simulink model "TST_EISGov_Governor"  (R2016b)
settings: Solver=FixedStepDiscrete  StartTime=0.0  StopTime=simTime  FixedStep=sampleTime  RelTol=1e-3
values from neighbouring files (symbols this model uses):
  testCase = 1    [initTST_EISGov_Governor_001.m]    (also in initTST_EISGov_Governor_002.m = 2; initTST_EISGov_Governor_003.m = 3; initTST_EISGov_Governor_004.m = 4; initTST_EISGov_Governor_005.m = 5)
libraries: simulink x43, UnitTest_Lib x36
(part 3 of 4)

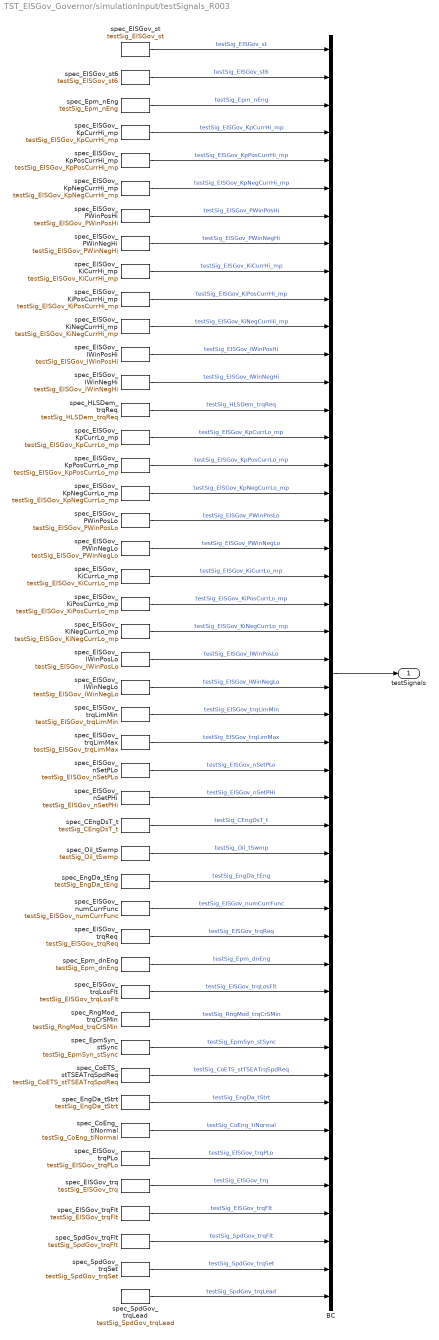
== system TST_EISGov_Governor/simulationInput/testSignals_R003 ==
  BC : BusCreator  Inputs=46
  spec_CEngDsT_t : FromWorkspace  VariableName=testSig_CEngDsT_t  Interpolate=off  OutputAfterFinalValue=Holding final value
  spec_CoETS_stTSEATrqSpdReq : FromWorkspace  VariableName=testSig_CoETS_stTSEATrqSpdReq  Interpolate=off  OutputAfterFinalValue=Holding final value
  spec_CoEng_tiNormal : FromWorkspace  VariableName=testSig_CoEng_tiNormal  Interpolate=off  OutputAfterFinalValue=Holding final value
  spec_EISGov_IWinNegHi : FromWorkspace  VariableName=testSig_EISGov_IWinNegHi  Interpolate=off  OutputAfterFinalValue=Holding final value
  spec_EISGov_IWinNegLo : FromWorkspace  VariableName=testSig_EISGov_IWinNegLo  Interpolate=off  OutputAfterFinalValue=Holding final value
  spec_EISGov_IWinPosHi : FromWorkspace  VariableName=testSig_EISGov_IWinPosHi  Interpolate=off  OutputAfterFinalValue=Holding final value
  spec_EISGov_IWinPosLo : FromWorkspace  VariableName=testSig_EISGov_IWinPosLo  Interpolate=off  OutputAfterFinalValue=Holding final value
  spec_EISGov_KiCurrHi_mp : FromWorkspace  VariableName=testSig_EISGov_KiCurrHi_mp  Interpolate=off  OutputAfterFinalValue=Holding final value
  spec_EISGov_KiCurrLo_mp : FromWorkspace  VariableName=testSig_EISGov_KiCurrLo_mp  Interpolate=off  OutputAfterFinalValue=Holding final value
  spec_EISGov_KiNegCurrHi_mp : FromWorkspace  VariableName=testSig_EISGov_KiNegCurrHi_mp  Interpolate=off  OutputAfterFinalValue=Holding final value
  spec_EISGov_KiNegCurrLo_mp : FromWorkspace  VariableName=testSig_EISGov_KiNegCurrLo_mp  Interpolate=off  OutputAfterFinalValue=Holding final value
  spec_EISGov_KiPosCurrHi_mp : FromWorkspace  VariableName=testSig_EISGov_KiPosCurrHi_mp  Interpolate=off  OutputAfterFinalValue=Holding final value
  spec_EISGov_KiPosCurrLo_mp : FromWorkspace  VariableName=testSig_EISGov_KiPosCurrLo_mp  Interpolate=off  OutputAfterFinalValue=Holding final value
  spec_EISGov_KpCurrHi_mp : FromWorkspace  VariableName=testSig_EISGov_KpCurrHi_mp  Interpolate=off  OutputAfterFinalValue=Holding final value
  spec_EISGov_KpCurrLo_mp : FromWorkspace  VariableName=testSig_EISGov_KpCurrLo_mp  Interpolate=off  OutputAfterFinalValue=Holding final value
  spec_EISGov_KpNegCurrHi_mp : FromWorkspace  VariableName=testSig_EISGov_KpNegCurrHi_mp  Interpolate=off  OutputAfterFinalValue=Holding final value
  spec_EISGov_KpNegCurrLo_mp : FromWorkspace  VariableName=testSig_EISGov_KpNegCurrLo_mp  Interpolate=off  OutputAfterFinalValue=Holding final value
  spec_EISGov_KpPosCurrHi_mp : FromWorkspace  VariableName=testSig_EISGov_KpPosCurrHi_mp  Interpolate=off  OutputAfterFinalValue=Holding final value
  spec_EISGov_KpPosCurrLo_mp : FromWorkspace  VariableName=testSig_EISGov_KpPosCurrLo_mp  Interpolate=off  OutputAfterFinalValue=Holding final value
  spec_EISGov_PWinNegHi : FromWorkspace  VariableName=testSig_EISGov_PWinNegHi  Interpolate=off  OutputAfterFinalValue=Holding final value
  spec_EISGov_PWinNegLo : FromWorkspace  VariableName=testSig_EISGov_PWinNegLo  Interpolate=off  OutputAfterFinalValue=Holding final value
  spec_EISGov_PWinPosHi : FromWorkspace  VariableName=testSig_EISGov_PWinPosHi  Interpolate=off  OutputAfterFinalValue=Holding final value
  spec_EISGov_PWinPosLo : FromWorkspace  VariableName=testSig_EISGov_PWinPosLo  Interpolate=off  OutputAfterFinalValue=Holding final value
  spec_EISGov_nSetPHi : FromWorkspace  VariableName=testSig_EISGov_nSetPHi  Interpolate=off  OutputAfterFinalValue=Holding final value
  spec_EISGov_nSetPLo : FromWorkspace  VariableName=testSig_EISGov_nSetPLo  Interpolate=off  OutputAfterFinalValue=Holding final value
  spec_EISGov_numCurrFunc : FromWorkspace  VariableName=testSig_EISGov_numCurrFunc  Interpolate=off  OutputAfterFinalValue=Holding final value
  spec_EISGov_st : FromWorkspace  VariableName=testSig_EISGov_st  Interpolate=off  OutputAfterFinalValue=Holding final value
  spec_EISGov_st6 : FromWorkspace  VariableName=testSig_EISGov_st6  Interpolate=off  OutputAfterFinalValue=Holding final value
  spec_EISGov_trq : FromWorkspace  VariableName=testSig_EISGov_trq  Interpolate=off  OutputAfterFinalValue=Holding final value
  spec_EISGov_trqFlt : FromWorkspace  VariableName=testSig_EISGov_trqFlt  Interpolate=off  OutputAfterFinalValue=Holding final value
  spec_EISGov_trqLimMax : FromWorkspace  VariableName=testSig_EISGov_trqLimMax  Interpolate=off  OutputAfterFinalValue=Holding final value
  spec_EISGov_trqLimMin : FromWorkspace  VariableName=testSig_EISGov_trqLimMin  Interpolate=off  OutputAfterFinalValue=Holding final value
  spec_EISGov_trqLosFlt : FromWorkspace  VariableName=testSig_EISGov_trqLosFlt  Interpolate=off  OutputAfterFinalValue=Holding final value
  spec_EISGov_trqPLo : FromWorkspace  VariableName=testSig_EISGov_trqPLo  Interpolate=off  OutputAfterFinalValue=Holding final value
  spec_EISGov_trqReq : FromWorkspace  VariableName=testSig_EISGov_trqReq  Interpolate=off  OutputAfterFinalValue=Holding final value
  spec_EngDa_tEng : FromWorkspace  VariableName=testSig_EngDa_tEng  Interpolate=off  OutputAfterFinalValue=Holding final value
  spec_EngDa_tStrt : FromWorkspace  VariableName=testSig_EngDa_tStrt  Interpolate=off  OutputAfterFinalValue=Holding final value
  spec_EpmSyn_stSync : FromWorkspace  VariableName=testSig_EpmSyn_stSync  Interpolate=off  OutputAfterFinalValue=Holding final value
  spec_Epm_dnEng : FromWorkspace  VariableName=testSig_Epm_dnEng  Interpolate=off  OutputAfterFinalValue=Holding final value
  spec_Epm_nEng : FromWorkspace  VariableName=testSig_Epm_nEng  Interpolate=off  OutputAfterFinalValue=Holding final value
  spec_HLSDem_trqReq : FromWorkspace  VariableName=testSig_HLSDem_trqReq  Interpolate=off  OutputAfterFinalValue=Holding final value
  spec_Oil_tSwmp : FromWorkspace  VariableName=testSig_Oil_tSwmp  Interpolate=off  OutputAfterFinalValue=Holding final value
  spec_RngMod_trqCrSMin : FromWorkspace  VariableName=testSig_RngMod_trqCrSMin  Interpolate=off  OutputAfterFinalValue=Holding final value
  spec_SpdGov_trqFlt : FromWorkspace  VariableName=testSig_SpdGov_trqFlt  Interpolate=off  OutputAfterFinalValue=Holding final value
  spec_SpdGov_trqLead : FromWorkspace  VariableName=testSig_SpdGov_trqLead  Interpolate=off  OutputAfterFinalValue=Holding final value
  spec_SpdGov_trqSet : FromWorkspace  VariableName=testSig_SpdGov_trqSet  Interpolate=off  OutputAfterFinalValue=Holding final value
  testSignals : Outport
  wires:
  BC/1 -> testSignals/1
  spec_EISGov_st/1 -> BC/1  "testSig_EISGov_st"
  spec_EISGov_st6/1 -> BC/2  "testSig_EISGov_st6"
  spec_Epm_nEng/1 -> BC/3  "testSig_Epm_nEng"
  spec_EISGov_KpCurrHi_mp/1 -> BC/4  "testSig_EISGov_KpCurrHi_mp"
  spec_EISGov_KpPosCurrHi_mp/1 -> BC/5  "testSig_EISGov_KpPosCurrHi_mp"
  spec_EISGov_KpNegCurrHi_mp/1 -> BC/6  "testSig_EISGov_KpNegCurrHi_mp"
  spec_EISGov_PWinPosHi/1 -> BC/7  "testSig_EISGov_PWinPosHi"
  spec_EISGov_PWinNegHi/1 -> BC/8  "testSig_EISGov_PWinNegHi"
  spec_EISGov_KiCurrHi_mp/1 -> BC/9  "testSig_EISGov_KiCurrHi_mp"
  spec_EISGov_KiPosCurrHi_mp/1 -> BC/10  "testSig_EISGov_KiPosCurrHi_mp"
  spec_EISGov_KiNegCurrHi_mp/1 -> BC/11  "testSig_EISGov_KiNegCurrHi_mp"
  spec_EISGov_IWinPosHi/1 -> BC/12  "testSig_EISGov_IWinPosHi"
  spec_EISGov_IWinNegHi/1 -> BC/13  "testSig_EISGov_IWinNegHi"
  spec_HLSDem_trqReq/1 -> BC/14  "testSig_HLSDem_trqReq"
  spec_EISGov_KpCurrLo_mp/1 -> BC/15  "testSig_EISGov_KpCurrLo_mp"
  spec_EISGov_KpPosCurrLo_mp/1 -> BC/16  "testSig_EISGov_KpPosCurrLo_mp"
  spec_EISGov_KpNegCurrLo_mp/1 -> BC/17  "testSig_EISGov_KpNegCurrLo_mp"
  spec_EISGov_PWinPosLo/1 -> BC/18  "testSig_EISGov_PWinPosLo"
  spec_EISGov_PWinNegLo/1 -> BC/19  "testSig_EISGov_PWinNegLo"
  spec_EISGov_KiCurrLo_mp/1 -> BC/20  "testSig_EISGov_KiCurrLo_mp"
  spec_EISGov_KiPosCurrLo_mp/1 -> BC/21  "testSig_EISGov_KiPosCurrLo_mp"
  spec_EISGov_KiNegCurrLo_mp/1 -> BC/22  "testSig_EISGov_KiNegCurrLo_mp"
  spec_EISGov_IWinPosLo/1 -> BC/23  "testSig_EISGov_IWinPosLo"
  spec_EISGov_IWinNegLo/1 -> BC/24  "testSig_EISGov_IWinNegLo"
  spec_EISGov_trqLimMin/1 -> BC/25  "testSig_EISGov_trqLimMin"
  spec_EISGov_trqLimMax/1 -> BC/26  "testSig_EISGov_trqLimMax"
  spec_EISGov_nSetPLo/1 -> BC/27  "testSig_EISGov_nSetPLo"
  spec_EISGov_nSetPHi/1 -> BC/28  "testSig_EISGov_nSetPHi"
  spec_CEngDsT_t/1 -> BC/29  "testSig_CEngDsT_t"
  spec_Oil_tSwmp/1 -> BC/30  "testSig_Oil_tSwmp"
  spec_EngDa_tEng/1 -> BC/31  "testSig_EngDa_tEng"
  spec_EISGov_numCurrFunc/1 -> BC/32  "testSig_EISGov_numCurrFunc"
  spec_EISGov_trqReq/1 -> BC/33  "testSig_EISGov_trqReq"
  spec_Epm_dnEng/1 -> BC/34  "testSig_Epm_dnEng"
  spec_EISGov_trqLosFlt/1 -> BC/35  "testSig_EISGov_trqLosFlt"
  spec_RngMod_trqCrSMin/1 -> BC/36  "testSig_RngMod_trqCrSMin"
  spec_EpmSyn_stSync/1 -> BC/37  "testSig_EpmSyn_stSync"
  spec_CoETS_stTSEATrqSpdReq/1 -> BC/38  "testSig_CoETS_stTSEATrqSpdReq"
  spec_EngDa_tStrt/1 -> BC/39  "testSig_EngDa_tStrt"
  spec_CoEng_tiNormal/1 -> BC/40  "testSig_CoEng_tiNormal"
  spec_EISGov_trqPLo/1 -> BC/41  "testSig_EISGov_trqPLo"
  spec_EISGov_trq/1 -> BC/42  "testSig_EISGov_trq"
  spec_EISGov_trqFlt/1 -> BC/43  "testSig_EISGov_trqFlt"
  spec_SpdGov_trqFlt/1 -> BC/44  "testSig_SpdGov_trqFlt"
  spec_SpdGov_trqSet/1 -> BC/45  "testSig_SpdGov_trqSet"
  spec_SpdGov_trqLead/1 -> BC/46  "testSig_SpdGov_trqLead"

== system TST_EISGov_Governor/simulationInput/testSignals_R004 ==
  BC : BusCreator  Inputs=46
  spec_CEngDsT_t : FromWorkspace  VariableName=testSig_CEngDsT_t  Interpolate=off  OutputAfterFinalValue=Holding final value
  spec_CoETS_stTSEATrqSpdReq : FromWorkspace  VariableName=testSig_CoETS_stTSEATrqSpdReq  Interpolate=off  OutputAfterFinalValue=Holding final value
  spec_CoEng_tiNormal : FromWorkspace  VariableName=testSig_CoEng_tiNormal  Interpolate=off  OutputAfterFinalValue=Holding final value
  spec_EISGov_IWinNegHi : FromWorkspace  VariableName=testSig_EISGov_IWinNegHi  Interpolate=off  OutputAfterFinalValue=Holding final value
  spec_EISGov_IWinNegLo : FromWorkspace  VariableName=testSig_EISGov_IWinNegLo  Interpolate=off  OutputAfterFinalValue=Holding final value
  spec_EISGov_IWinPosHi : FromWorkspace  VariableName=testSig_EISGov_IWinPosHi  Interpolate=off  OutputAfterFinalValue=Holding final value
  spec_EISGov_IWinPosLo : FromWorkspace  VariableName=testSig_EISGov_IWinPosLo  Interpolate=off  OutputAfterFinalValue=Holding final value
  spec_EISGov_KiCurrHi_mp : FromWorkspace  VariableName=testSig_EISGov_KiCurrHi_mp  Interpolate=off  OutputAfterFinalValue=Holding final value
  spec_EISGov_KiCurrLo_mp : FromWorkspace  VariableName=testSig_EISGov_KiCurrLo_mp  Interpolate=off  OutputAfterFinalValue=Holding final value
  spec_EISGov_KiNegCurrHi_mp : FromWorkspace  VariableName=testSig_EISGov_KiNegCurrHi_mp  Interpolate=off  OutputAfterFinalValue=Holding final value
  spec_EISGov_KiNegCurrLo_mp : FromWorkspace  VariableName=testSig_EISGov_KiNegCurrLo_mp  Interpolate=off  OutputAfterFinalValue=Holding final value
  spec_EISGov_KiPosCurrHi_mp : FromWorkspace  VariableName=testSig_EISGov_KiPosCurrHi_mp  Interpolate=off  OutputAfterFinalValue=Holding final value
  spec_EISGov_KiPosCurrLo_mp : FromWorkspace  VariableName=testSig_EISGov_KiPosCurrLo_mp  Interpolate=off  OutputAfterFinalValue=Holding final value
  spec_EISGov_KpCurrHi_mp : FromWorkspace  VariableName=testSig_EISGov_KpCurrHi_mp  Interpolate=off  OutputAfterFinalValue=Holding final value
  spec_EISGov_KpCurrLo_mp : FromWorkspace  VariableName=testSig_EISGov_KpCurrLo_mp  Interpolate=off  OutputAfterFinalValue=Holding final value
  spec_EISGov_KpNegCurrHi_mp : FromWorkspace  VariableName=testSig_EISGov_KpNegCurrHi_mp  Interpolate=off  OutputAfterFinalValue=Holding final value
  spec_EISGov_KpNegCurrLo_mp : FromWorkspace  VariableName=testSig_EISGov_KpNegCurrLo_mp  Interpolate=off  OutputAfterFinalValue=Holding final value
  spec_EISGov_KpPosCurrHi_mp : FromWorkspace  VariableName=testSig_EISGov_KpPosCurrHi_mp  Interpolate=off  OutputAfterFinalValue=Holding final value
  spec_EISGov_KpPosCurrLo_mp : FromWorkspace  VariableName=testSig_EISGov_KpPosCurrLo_mp  Interpolate=off  OutputAfterFinalValue=Holding final value
  spec_EISGov_PWinNegHi : FromWorkspace  VariableName=testSig_EISGov_PWinNegHi  Interpolate=off  OutputAfterFinalValue=Holding final value
  spec_EISGov_PWinNegLo : FromWorkspace  VariableName=testSig_EISGov_PWinNegLo  Interpolate=off  OutputAfterFinalValue=Holding final value
  spec_EISGov_PWinPosHi : FromWorkspace  VariableName=testSig_EISGov_PWinPosHi  Interpolate=off  OutputAfterFinalValue=Holding final value
  spec_EISGov_PWinPosLo : FromWorkspace  VariableName=testSig_EISGov_PWinPosLo  Interpolate=off  OutputAfterFinalValue=Holding final value
  spec_EISGov_nSetPHi : FromWorkspace  VariableName=testSig_EISGov_nSetPHi  Interpolate=off  OutputAfterFinalValue=Holding final value
  spec_EISGov_nSetPLo : FromWorkspace  VariableName=testSig_EISGov_nSetPLo  Interpolate=off  OutputAfterFinalValue=Holding final value
  spec_EISGov_numCurrFunc : FromWorkspace  VariableName=testSig_EISGov_numCurrFunc  Interpolate=off  OutputAfterFinalValue=Holding final value
  spec_EISGov_st : FromWorkspace  VariableName=testSig_EISGov_st  Interpolate=off  OutputAfterFinalValue=Holding final value
  spec_EISGov_st6 : FromWorkspace  VariableName=testSig_EISGov_st6  Interpolate=off  OutputAfterFinalValue=Holding final value
  spec_EISGov_trq : FromWorkspace  VariableName=testSig_EISGov_trq  Interpolate=off  OutputAfterFinalValue=Holding final value
  spec_EISGov_trqFlt : FromWorkspace  VariableName=testSig_EISGov_trqFlt  Interpolate=off  OutputAfterFinalValue=Holding final value
  spec_EISGov_trqLimMax : FromWorkspace  VariableName=testSig_EISGov_trqLimMax  Interpolate=off  OutputAfterFinalValue=Holding final value
  spec_EISGov_trqLimMin : FromWorkspace  VariableName=testSig_EISGov_trqLimMin  Interpolate=off  OutputAfterFinalValue=Holding final value
  spec_EISGov_trqLosFlt : FromWorkspace  VariableName=testSig_EISGov_trqLosFlt  Interpolate=off  OutputAfterFinalValue=Holding final value
  spec_EISGov_trqPLo : FromWorkspace  VariableName=testSig_EISGov_trqPLo  Interpolate=off  OutputAfterFinalValue=Holding final value
  spec_EISGov_trqReq : FromWorkspace  VariableName=testSig_EISGov_trqReq  Interpolate=off  OutputAfterFinalValue=Holding final value
  spec_EngDa_tEng : FromWorkspace  VariableName=testSig_EngDa_tEng  Interpolate=off  OutputAfterFinalValue=Holding final value
  spec_EngDa_tStrt : FromWorkspace  VariableName=testSig_EngDa_tStrt  Interpolate=off  OutputAfterFinalValue=Holding final value
  spec_EpmSyn_stSync : FromWorkspace  VariableName=testSig_EpmSyn_stSync  Interpolate=off  OutputAfterFinalValue=Holding final value
  spec_Epm_dnEng : FromWorkspace  VariableName=testSig_Epm_dnEng  Interpolate=off  OutputAfterFinalValue=Holding final value
  spec_Epm_nEng : FromWorkspace  VariableName=testSig_Epm_nEng  Interpolate=off  OutputAfterFinalValue=Holding final value
  spec_HLSDem_trqReq : FromWorkspace  VariableName=testSig_HLSDem_trqReq  Interpolate=off  OutputAfterFinalValue=Holding final value
  spec_Oil_tSwmp : FromWorkspace  VariableName=testSig_Oil_tSwmp  Interpolate=off  OutputAfterFinalValue=Holding final value
  spec_RngMod_trqCrSMin : FromWorkspace  VariableName=testSig_RngMod_trqCrSMin  Interpolate=off  OutputAfterFinalValue=Holding final value
  spec_SpdGov_trqFlt : FromWorkspace  VariableName=testSig_SpdGov_trqFlt  Interpolate=off  OutputAfterFinalValue=Holding final value
  spec_SpdGov_trqLead : FromWorkspace  VariableName=testSig_SpdGov_trqLead  Interpolate=off  OutputAfterFinalValue=Holding final value
  spec_SpdGov_trqSet : FromWorkspace  VariableName=testSig_SpdGov_trqSet  Interpolate=off  OutputAfterFinalValue=Holding final value
  testSignals : Outport
  wires:
  BC/1 -> testSignals/1
  spec_EISGov_st/1 -> BC/1  "testSig_EISGov_st"
  spec_EISGov_st6/1 -> BC/2  "testSig_EISGov_st6"
  spec_Epm_nEng/1 -> BC/3  "testSig_Epm_nEng"
  spec_EISGov_KpCurrHi_mp/1 -> BC/4  "testSig_EISGov_KpCurrHi_mp"
  spec_EISGov_KpPosCurrHi_mp/1 -> BC/5  "testSig_EISGov_KpPosCurrHi_mp"
  spec_EISGov_KpNegCurrHi_mp/1 -> BC/6  "testSig_EISGov_KpNegCurrHi_mp"
  spec_EISGov_PWinPosHi/1 -> BC/7  "testSig_EISGov_PWinPosHi"
  spec_EISGov_PWinNegHi/1 -> BC/8  "testSig_EISGov_PWinNegHi"
  spec_EISGov_KiCurrHi_mp/1 -> BC/9  "testSig_EISGov_KiCurrHi_mp"
  spec_EISGov_KiPosCurrHi_mp/1 -> BC/10  "testSig_EISGov_KiPosCurrHi_mp"
  spec_EISGov_KiNegCurrHi_mp/1 -> BC/11  "testSig_EISGov_KiNegCurrHi_mp"
  spec_EISGov_IWinPosHi/1 -> BC/12  "testSig_EISGov_IWinPosHi"
  spec_EISGov_IWinNegHi/1 -> BC/13  "testSig_EISGov_IWinNegHi"
  spec_HLSDem_trqReq/1 -> BC/14  "testSig_HLSDem_trqReq"
  spec_EISGov_KpCurrLo_mp/1 -> BC/15  "testSig_EISGov_KpCurrLo_mp"
  spec_EISGov_KpPosCurrLo_mp/1 -> BC/16  "testSig_EISGov_KpPosCurrLo_mp"
  spec_EISGov_KpNegCurrLo_mp/1 -> BC/17  "testSig_EISGov_KpNegCurrLo_mp"
  spec_EISGov_PWinPosLo/1 -> BC/18  "testSig_EISGov_PWinPosLo"
  spec_EISGov_PWinNegLo/1 -> BC/19  "testSig_EISGov_PWinNegLo"
  spec_EISGov_KiCurrLo_mp/1 -> BC/20  "testSig_EISGov_KiCurrLo_mp"
  spec_EISGov_KiPosCurrLo_mp/1 -> BC/21  "testSig_EISGov_KiPosCurrLo_mp"
  spec_EISGov_KiNegCurrLo_mp/1 -> BC/22  "testSig_EISGov_KiNegCurrLo_mp"
  spec_EISGov_IWinPosLo/1 -> BC/23  "testSig_EISGov_IWinPosLo"
  spec_EISGov_IWinNegLo/1 -> BC/24  "testSig_EISGov_IWinNegLo"
  spec_EISGov_trqLimMin/1 -> BC/25  "testSig_EISGov_trqLimMin"
  spec_EISGov_trqLimMax/1 -> BC/26  "testSig_EISGov_trqLimMax"
  spec_EISGov_nSetPLo/1 -> BC/27  "testSig_EISGov_nSetPLo"
  spec_EISGov_nSetPHi/1 -> BC/28  "testSig_EISGov_nSetPHi"
  spec_CEngDsT_t/1 -> BC/29  "testSig_CEngDsT_t"
  spec_Oil_tSwmp/1 -> BC/30  "testSig_Oil_tSwmp"
  spec_EngDa_tEng/1 -> BC/31  "testSig_EngDa_tEng"
  spec_EISGov_numCurrFunc/1 -> BC/32  "testSig_EISGov_numCurrFunc"
  spec_EISGov_trqReq/1 -> BC/33  "testSig_EISGov_trqReq"
  spec_Epm_dnEng/1 -> BC/34  "testSig_Epm_dnEng"
  spec_EISGov_trqLosFlt/1 -> BC/35  "testSig_EISGov_trqLosFlt"
  spec_RngMod_trqCrSMin/1 -> BC/36  "testSig_RngMod_trqCrSMin"
  spec_EpmSyn_stSync/1 -> BC/37  "testSig_EpmSyn_stSync"
  spec_CoETS_stTSEATrqSpdReq/1 -> BC/38  "testSig_CoETS_stTSEATrqSpdReq"
  spec_EngDa_tStrt/1 -> BC/39  "testSig_EngDa_tStrt"
  spec_CoEng_tiNormal/1 -> BC/40  "testSig_CoEng_tiNormal"
  spec_EISGov_trqPLo/1 -> BC/41  "testSig_EISGov_trqPLo"
  spec_EISGov_trq/1 -> BC/42  "testSig_EISGov_trq"
  spec_EISGov_trqFlt/1 -> BC/43  "testSig_EISGov_trqFlt"
  spec_SpdGov_trqFlt/1 -> BC/44  "testSig_SpdGov_trqFlt"
  spec_SpdGov_trqSet/1 -> BC/45  "testSig_SpdGov_trqSet"
  spec_SpdGov_trqLead/1 -> BC/46  "testSig_SpdGov_trqLead"

== system TST_EISGov_Governor/simulationInput/testSignals_R005 ==
  BC : BusCreator  Inputs=46
  spec_CEngDsT_t : FromWorkspace  VariableName=testSig_CEngDsT_t  Interpolate=off  OutputAfterFinalValue=Holding final value
  spec_CoETS_stTSEATrqSpdReq : FromWorkspace  VariableName=testSig_CoETS_stTSEATrqSpdReq  Interpolate=off  OutputAfterFinalValue=Holding final value
  spec_CoEng_tiNormal : FromWorkspace  VariableName=testSig_CoEng_tiNormal  Interpolate=off  OutputAfterFinalValue=Holding final value
  spec_EISGov_IWinNegHi : FromWorkspace  VariableName=testSig_EISGov_IWinNegHi  Interpolate=off  OutputAfterFinalValue=Holding final value
  spec_EISGov_IWinNegLo : FromWorkspace  VariableName=testSig_EISGov_IWinNegLo  Interpolate=off  OutputAfterFinalValue=Holding final value
  spec_EISGov_IWinPosHi : FromWorkspace  VariableName=testSig_EISGov_IWinPosHi  Interpolate=off  OutputAfterFinalValue=Holding final value
  spec_EISGov_IWinPosLo : FromWorkspace  VariableName=testSig_EISGov_IWinPosLo  Interpolate=off  OutputAfterFinalValue=Holding final value
  spec_EISGov_KiCurrHi_mp : FromWorkspace  VariableName=testSig_EISGov_KiCurrHi_mp  Interpolate=off  OutputAfterFinalValue=Holding final value
  spec_EISGov_KiCurrLo_mp : FromWorkspace  VariableName=testSig_EISGov_KiCurrLo_mp  Interpolate=off  OutputAfterFinalValue=Holding final value
  spec_EISGov_KiNegCurrHi_mp : FromWorkspace  VariableName=testSig_EISGov_KiNegCurrHi_mp  Interpolate=off  OutputAfterFinalValue=Holding final value
  spec_EISGov_KiNegCurrLo_mp : FromWorkspace  VariableName=testSig_EISGov_KiNegCurrLo_mp  Interpolate=off  OutputAfterFinalValue=Holding final value
  spec_EISGov_KiPosCurrHi_mp : FromWorkspace  VariableName=testSig_EISGov_KiPosCurrHi_mp  Interpolate=off  OutputAfterFinalValue=Holding final value
  spec_EISGov_KiPosCurrLo_mp : FromWorkspace  VariableName=testSig_EISGov_KiPosCurrLo_mp  Interpolate=off  OutputAfterFinalValue=Holding final value
  spec_EISGov_KpCurrHi_mp : FromWorkspace  VariableName=testSig_EISGov_KpCurrHi_mp  Interpolate=off  OutputAfterFinalValue=Holding final value
  spec_EISGov_KpCurrLo_mp : FromWorkspace  VariableName=testSig_EISGov_KpCurrLo_mp  Interpolate=off  OutputAfterFinalValue=Holding final value
  spec_EISGov_KpNegCurrHi_mp : FromWorkspace  VariableName=testSig_EISGov_KpNegCurrHi_mp  Interpolate=off  OutputAfterFinalValue=Holding final value
  spec_EISGov_KpNegCurrLo_mp : FromWorkspace  VariableName=testSig_EISGov_KpNegCurrLo_mp  Interpolate=off  OutputAfterFinalValue=Holding final value
  spec_EISGov_KpPosCurrHi_mp : FromWorkspace  VariableName=testSig_EISGov_KpPosCurrHi_mp  Interpolate=off  OutputAfterFinalValue=Holding final value
  spec_EISGov_KpPosCurrLo_mp : FromWorkspace  VariableName=testSig_EISGov_KpPosCurrLo_mp  Interpolate=off  OutputAfterFinalValue=Holding final value
  spec_EISGov_PWinNegHi : FromWorkspace  VariableName=testSig_EISGov_PWinNegHi  Interpolate=off  OutputAfterFinalValue=Holding final value
  spec_EISGov_PWinNegLo : FromWorkspace  VariableName=testSig_EISGov_PWinNegLo  Interpolate=off  OutputAfterFinalValue=Holding final value
  spec_EISGov_PWinPosHi : FromWorkspace  VariableName=testSig_EISGov_PWinPosHi  Interpolate=off  OutputAfterFinalValue=Holding final value
  spec_EISGov_PWinPosLo : FromWorkspace  VariableName=testSig_EISGov_PWinPosLo  Interpolate=off  OutputAfterFinalValue=Holding final value
  spec_EISGov_nSetPHi : FromWorkspace  VariableName=testSig_EISGov_nSetPHi  Interpolate=off  OutputAfterFinalValue=Holding final value
  spec_EISGov_nSetPLo : FromWorkspace  VariableName=testSig_EISGov_nSetPLo  Interpolate=off  OutputAfterFinalValue=Holding final value
  spec_EISGov_numCurrFunc : FromWorkspace  VariableName=testSig_EISGov_numCurrFunc  Interpolate=off  OutputAfterFinalValue=Holding final value
  spec_EISGov_st : FromWorkspace  VariableName=testSig_EISGov_st  Interpolate=off  OutputAfterFinalValue=Holding final value
  spec_EISGov_st6 : FromWorkspace  VariableName=testSig_EISGov_st6  Interpolate=off  OutputAfterFinalValue=Holding final value
  spec_EISGov_trq : FromWorkspace  VariableName=testSig_EISGov_trq  Interpolate=off  OutputAfterFinalValue=Holding final value
  spec_EISGov_trqFlt : FromWorkspace  VariableName=testSig_EISGov_trqFlt  Interpolate=off  OutputAfterFinalValue=Holding final value
  spec_EISGov_trqLimMax : FromWorkspace  VariableName=testSig_EISGov_trqLimMax  Interpolate=off  OutputAfterFinalValue=Holding final value
  spec_EISGov_trqLimMin : FromWorkspace  VariableName=testSig_EISGov_trqLimMin  Interpolate=off  OutputAfterFinalValue=Holding final value
  spec_EISGov_trqLosFlt : FromWorkspace  VariableName=testSig_EISGov_trqLosFlt  Interpolate=off  OutputAfterFinalValue=Holding final value
  spec_EISGov_trqPLo : FromWorkspace  VariableName=testSig_EISGov_trqPLo  Interpolate=off  OutputAfterFinalValue=Holding final value
  spec_EISGov_trqReq : FromWorkspace  VariableName=testSig_EISGov_trqReq  Interpolate=off  OutputAfterFinalValue=Holding final value
  spec_EngDa_tEng : FromWorkspace  VariableName=testSig_EngDa_tEng  Interpolate=off  OutputAfterFinalValue=Holding final value
  spec_EngDa_tStrt : FromWorkspace  VariableName=testSig_EngDa_tStrt  Interpolate=off  OutputAfterFinalValue=Holding final value
  spec_EpmSyn_stSync : FromWorkspace  VariableName=testSig_EpmSyn_stSync  Interpolate=off  OutputAfterFinalValue=Holding final value
  spec_Epm_dnEng : FromWorkspace  VariableName=testSig_Epm_dnEng  Interpolate=off  OutputAfterFinalValue=Holding final value
  spec_Epm_nEng : FromWorkspace  VariableName=testSig_Epm_nEng  Interpolate=off  OutputAfterFinalValue=Holding final value
  spec_HLSDem_trqReq : FromWorkspace  VariableName=testSig_HLSDem_trqReq  Interpolate=off  OutputAfterFinalValue=Holding final value
  spec_Oil_tSwmp : FromWorkspace  VariableName=testSig_Oil_tSwmp  Interpolate=off  OutputAfterFinalValue=Holding final value
  spec_RngMod_trqCrSMin : FromWorkspace  VariableName=testSig_RngMod_trqCrSMin  Interpolate=off  OutputAfterFinalValue=Holding final value
  spec_SpdGov_trqFlt : FromWorkspace  VariableName=testSig_SpdGov_trqFlt  Interpolate=off  OutputAfterFinalValue=Holding final value
  spec_SpdGov_trqLead : FromWorkspace  VariableName=testSig_SpdGov_trqLead  Interpolate=off  OutputAfterFinalValue=Holding final value
  spec_SpdGov_trqSet : FromWorkspace  VariableName=testSig_SpdGov_trqSet  Interpolate=off  OutputAfterFinalValue=Holding final value
  testSignals : Outport
  wires:
  BC/1 -> testSignals/1
  spec_EISGov_st/1 -> BC/1  "testSig_EISGov_st"
  spec_EISGov_st6/1 -> BC/2  "testSig_EISGov_st6"
  spec_Epm_nEng/1 -> BC/3  "testSig_Epm_nEng"
  spec_EISGov_KpCurrHi_mp/1 -> BC/4  "testSig_EISGov_KpCurrHi_mp"
  spec_EISGov_KpPosCurrHi_mp/1 -> BC/5  "testSig_EISGov_KpPosCurrHi_mp"
  spec_EISGov_KpNegCurrHi_mp/1 -> BC/6  "testSig_EISGov_KpNegCurrHi_mp"
  spec_EISGov_PWinPosHi/1 -> BC/7  "testSig_EISGov_PWinPosHi"
  spec_EISGov_PWinNegHi/1 -> BC/8  "testSig_EISGov_PWinNegHi"
  spec_EISGov_KiCurrHi_mp/1 -> BC/9  "testSig_EISGov_KiCurrHi_mp"
  spec_EISGov_KiPosCurrHi_mp/1 -> BC/10  "testSig_EISGov_KiPosCurrHi_mp"
  spec_EISGov_KiNegCurrHi_mp/1 -> BC/11  "testSig_EISGov_KiNegCurrHi_mp"
  spec_EISGov_IWinPosHi/1 -> BC/12  "testSig_EISGov_IWinPosHi"
  spec_EISGov_IWinNegHi/1 -> BC/13  "testSig_EISGov_IWinNegHi"
  spec_HLSDem_trqReq/1 -> BC/14  "testSig_HLSDem_trqReq"
  spec_EISGov_KpCurrLo_mp/1 -> BC/15  "testSig_EISGov_KpCurrLo_mp"
  spec_EISGov_KpPosCurrLo_mp/1 -> BC/16  "testSig_EISGov_KpPosCurrLo_mp"
  spec_EISGov_KpNegCurrLo_mp/1 -> BC/17  "testSig_EISGov_KpNegCurrLo_mp"
  spec_EISGov_PWinPosLo/1 -> BC/18  "testSig_EISGov_PWinPosLo"
  spec_EISGov_PWinNegLo/1 -> BC/19  "testSig_EISGov_PWinNegLo"
  spec_EISGov_KiCurrLo_mp/1 -> BC/20  "testSig_EISGov_KiCurrLo_mp"
  spec_EISGov_KiPosCurrLo_mp/1 -> BC/21  "testSig_EISGov_KiPosCurrLo_mp"
  spec_EISGov_KiNegCurrLo_mp/1 -> BC/22  "testSig_EISGov_KiNegCurrLo_mp"
  spec_EISGov_IWinPosLo/1 -> BC/23  "testSig_EISGov_IWinPosLo"
  spec_EISGov_IWinNegLo/1 -> BC/24  "testSig_EISGov_IWinNegLo"
  spec_EISGov_trqLimMin/1 -> BC/25  "testSig_EISGov_trqLimMin"
  spec_EISGov_trqLimMax/1 -> BC/26  "testSig_EISGov_trqLimMax"
  spec_EISGov_nSetPLo/1 -> BC/27  "testSig_EISGov_nSetPLo"
  spec_EISGov_nSetPHi/1 -> BC/28  "testSig_EISGov_nSetPHi"
  spec_CEngDsT_t/1 -> BC/29  "testSig_CEngDsT_t"
  spec_Oil_tSwmp/1 -> BC/30  "testSig_Oil_tSwmp"
  spec_EngDa_tEng/1 -> BC/31  "testSig_EngDa_tEng"
  spec_EISGov_numCurrFunc/1 -> BC/32  "testSig_EISGov_numCurrFunc"
  spec_EISGov_trqReq/1 -> BC/33  "testSig_EISGov_trqReq"
  spec_Epm_dnEng/1 -> BC/34  "testSig_Epm_dnEng"
  spec_EISGov_trqLosFlt/1 -> BC/35  "testSig_EISGov_trqLosFlt"
  spec_RngMod_trqCrSMin/1 -> BC/36  "testSig_RngMod_trqCrSMin"
  spec_EpmSyn_stSync/1 -> BC/37  "testSig_EpmSyn_stSync"
  spec_CoETS_stTSEATrqSpdReq/1 -> BC/38  "testSig_CoETS_stTSEATrqSpdReq"
  spec_EngDa_tStrt/1 -> BC/39  "testSig_EngDa_tStrt"
  spec_CoEng_tiNormal/1 -> BC/40  "testSig_CoEng_tiNormal"
  spec_EISGov_trqPLo/1 -> BC/41  "testSig_EISGov_trqPLo"
  spec_EISGov_trq/1 -> BC/42  "testSig_EISGov_trq"
  spec_EISGov_trqFlt/1 -> BC/43  "testSig_EISGov_trqFlt"
  spec_SpdGov_trqFlt/1 -> BC/44  "testSig_SpdGov_trqFlt"
  spec_SpdGov_trqSet/1 -> BC/45  "testSig_SpdGov_trqSet"
  spec_SpdGov_trqLead/1 -> BC/46  "testSig_SpdGov_trqLead"

== system TST_EISGov_Governor/simulationInput/testSignals_R006 ==
  BC : BusCreator  Inputs=46
  spec_CEngDsT_t : FromWorkspace  VariableName=testSig_CEngDsT_t  Interpolate=off  OutputAfterFinalValue=Holding final value
  spec_CoETS_stTSEATrqSpdReq : FromWorkspace  VariableName=testSig_CoETS_stTSEATrqSpdReq  Interpolate=off  OutputAfterFinalValue=Holding final value
  spec_CoEng_tiNormal : FromWorkspace  VariableName=testSig_CoEng_tiNormal  Interpolate=off  OutputAfterFinalValue=Holding final value
  spec_EISGov_IWinNegHi : FromWorkspace  VariableName=testSig_EISGov_IWinNegHi  Interpolate=off  OutputAfterFinalValue=Holding final value
  spec_EISGov_IWinNegLo : FromWorkspace  VariableName=testSig_EISGov_IWinNegLo  Interpolate=off  OutputAfterFinalValue=Holding final value
  spec_EISGov_IWinPosHi : FromWorkspace  VariableName=testSig_EISGov_IWinPosHi  Interpolate=off  OutputAfterFinalValue=Holding final value
  spec_EISGov_IWinPosLo : FromWorkspace  VariableName=testSig_EISGov_IWinPosLo  Interpolate=off  OutputAfterFinalValue=Holding final value
  spec_EISGov_KiCurrHi_mp : FromWorkspace  VariableName=testSig_EISGov_KiCurrHi_mp  Interpolate=off  OutputAfterFinalValue=Holding final value
  spec_EISGov_KiCurrLo_mp : FromWorkspace  VariableName=testSig_EISGov_KiCurrLo_mp  Interpolate=off  OutputAfterFinalValue=Holding final value
  spec_EISGov_KiNegCurrHi_mp : FromWorkspace  VariableName=testSig_EISGov_KiNegCurrHi_mp  Interpolate=off  OutputAfterFinalValue=Holding final value
  spec_EISGov_KiNegCurrLo_mp : FromWorkspace  VariableName=testSig_EISGov_KiNegCurrLo_mp  Interpolate=off  OutputAfterFinalValue=Holding final value
  spec_EISGov_KiPosCurrHi_mp : FromWorkspace  VariableName=testSig_EISGov_KiPosCurrHi_mp  Interpolate=off  OutputAfterFinalValue=Holding final value
  spec_EISGov_KiPosCurrLo_mp : FromWorkspace  VariableName=testSig_EISGov_KiPosCurrLo_mp  Interpolate=off  OutputAfterFinalValue=Holding final value
  spec_EISGov_KpCurrHi_mp : FromWorkspace  VariableName=testSig_EISGov_KpCurrHi_mp  Interpolate=off  OutputAfterFinalValue=Holding final value
  spec_EISGov_KpCurrLo_mp : FromWorkspace  VariableName=testSig_EISGov_KpCurrLo_mp  Interpolate=off  OutputAfterFinalValue=Holding final value
  spec_EISGov_KpNegCurrHi_mp : FromWorkspace  VariableName=testSig_EISGov_KpNegCurrHi_mp  Interpolate=off  OutputAfterFinalValue=Holding final value
  spec_EISGov_KpNegCurrLo_mp : FromWorkspace  VariableName=testSig_EISGov_KpNegCurrLo_mp  Interpolate=off  OutputAfterFinalValue=Holding final value
  spec_EISGov_KpPosCurrHi_mp : FromWorkspace  VariableName=testSig_EISGov_KpPosCurrHi_mp  Interpolate=off  OutputAfterFinalValue=Holding final value
  spec_EISGov_KpPosCurrLo_mp : FromWorkspace  VariableName=testSig_EISGov_KpPosCurrLo_mp  Interpolate=off  OutputAfterFinalValue=Holding final value
  spec_EISGov_PWinNegHi : FromWorkspace  VariableName=testSig_EISGov_PWinNegHi  Interpolate=off  OutputAfterFinalValue=Holding final value
  spec_EISGov_PWinNegLo : FromWorkspace  VariableName=testSig_EISGov_PWinNegLo  Interpolate=off  OutputAfterFinalValue=Holding final value
  spec_EISGov_PWinPosHi : FromWorkspace  VariableName=testSig_EISGov_PWinPosHi  Interpolate=off  OutputAfterFinalValue=Holding final value
  spec_EISGov_PWinPosLo : FromWorkspace  VariableName=testSig_EISGov_PWinPosLo  Interpolate=off  OutputAfterFinalValue=Holding final value
  spec_EISGov_nSetPHi : FromWorkspace  VariableName=testSig_EISGov_nSetPHi  Interpolate=off  OutputAfterFinalValue=Holding final value
  spec_EISGov_nSetPLo : FromWorkspace  VariableName=testSig_EISGov_nSetPLo  Interpolate=off  OutputAfterFinalValue=Holding final value
  spec_EISGov_numCurrFunc : FromWorkspace  VariableName=testSig_EISGov_numCurrFunc  Interpolate=off  OutputAfterFinalValue=Holding final value
  spec_EISGov_st : FromWorkspace  VariableName=testSig_EISGov_st  Interpolate=off  OutputAfterFinalValue=Holding final value
  spec_EISGov_st6 : FromWorkspace  VariableName=testSig_EISGov_st6  Interpolate=off  OutputAfterFinalValue=Holding final value
  spec_EISGov_trq : FromWorkspace  VariableName=testSig_EISGov_trq  Interpolate=off  OutputAfterFinalValue=Holding final value
  spec_EISGov_trqFlt : FromWorkspace  VariableName=testSig_EISGov_trqFlt  Interpolate=off  OutputAfterFinalValue=Holding final value
  spec_EISGov_trqLimMax : FromWorkspace  VariableName=testSig_EISGov_trqLimMax  Interpolate=off  OutputAfterFinalValue=Holding final value
  spec_EISGov_trqLimMin : FromWorkspace  VariableName=testSig_EISGov_trqLimMin  Interpolate=off  OutputAfterFinalValue=Holding final value
  spec_EISGov_trqLosFlt : FromWorkspace  VariableName=testSig_EISGov_trqLosFlt  Interpolate=off  OutputAfterFinalValue=Holding final value
  spec_EISGov_trqPLo : FromWorkspace  VariableName=testSig_EISGov_trqPLo  Interpolate=off  OutputAfterFinalValue=Holding final value
  spec_EISGov_trqReq : FromWorkspace  VariableName=testSig_EISGov_trqReq  Interpolate=off  OutputAfterFinalValue=Holding final value
  spec_EngDa_tEng : FromWorkspace  VariableName=testSig_EngDa_tEng  Interpolate=off  OutputAfterFinalValue=Holding final value
  spec_EngDa_tStrt : FromWorkspace  VariableName=testSig_EngDa_tStrt  Interpolate=off  OutputAfterFinalValue=Holding final value
  spec_EpmSyn_stSync : FromWorkspace  VariableName=testSig_EpmSyn_stSync  Interpolate=off  OutputAfterFinalValue=Holding final value
  spec_Epm_dnEng : FromWorkspace  VariableName=testSig_Epm_dnEng  Interpolate=off  OutputAfterFinalValue=Holding final value
  spec_Epm_nEng : FromWorkspace  VariableName=testSig_Epm_nEng  Interpolate=off  OutputAfterFinalValue=Holding final value
  spec_HLSDem_trqReq : FromWorkspace  VariableName=testSig_HLSDem_trqReq  Interpolate=off  OutputAfterFinalValue=Holding final value
  spec_Oil_tSwmp : FromWorkspace  VariableName=testSig_Oil_tSwmp  Interpolate=off  OutputAfterFinalValue=Holding final value
  spec_RngMod_trqCrSMin : FromWorkspace  VariableName=testSig_RngMod_trqCrSMin  Interpolate=off  OutputAfterFinalValue=Holding final value
  spec_SpdGov_trqFlt : FromWorkspace  VariableName=testSig_SpdGov_trqFlt  Interpolate=off  OutputAfterFinalValue=Holding final value
  spec_SpdGov_trqLead : FromWorkspace  VariableName=testSig_SpdGov_trqLead  Interpolate=off  OutputAfterFinalValue=Holding final value
  spec_SpdGov_trqSet : FromWorkspace  VariableName=testSig_SpdGov_trqSet  Interpolate=off  OutputAfterFinalValue=Holding final value
  testSignals : Outport
  wires:
  BC/1 -> testSignals/1
  spec_EISGov_st/1 -> BC/1  "testSig_EISGov_st"
  spec_EISGov_st6/1 -> BC/2  "testSig_EISGov_st6"
  spec_Epm_nEng/1 -> BC/3  "testSig_Epm_nEng"
  spec_EISGov_KpCurrHi_mp/1 -> BC/4  "testSig_EISGov_KpCurrHi_mp"
  spec_EISGov_KpPosCurrHi_mp/1 -> BC/5  "testSig_EISGov_KpPosCurrHi_mp"
  spec_EISGov_KpNegCurrHi_mp/1 -> BC/6  "testSig_EISGov_KpNegCurrHi_mp"
  spec_EISGov_PWinPosHi/1 -> BC/7  "testSig_EISGov_PWinPosHi"
  spec_EISGov_PWinNegHi/1 -> BC/8  "testSig_EISGov_PWinNegHi"
  spec_EISGov_KiCurrHi_mp/1 -> BC/9  "testSig_EISGov_KiCurrHi_mp"
  spec_EISGov_KiPosCurrHi_mp/1 -> BC/10  "testSig_EISGov_KiPosCurrHi_mp"
  spec_EISGov_KiNegCurrHi_mp/1 -> BC/11  "testSig_EISGov_KiNegCurrHi_mp"
  spec_EISGov_IWinPosHi/1 -> BC/12  "testSig_EISGov_IWinPosHi"
  spec_EISGov_IWinNegHi/1 -> BC/13  "testSig_EISGov_IWinNegHi"
  spec_HLSDem_trqReq/1 -> BC/14  "testSig_HLSDem_trqReq"
  spec_EISGov_KpCurrLo_mp/1 -> BC/15  "testSig_EISGov_KpCurrLo_mp"
  spec_EISGov_KpPosCurrLo_mp/1 -> BC/16  "testSig_EISGov_KpPosCurrLo_mp"
  spec_EISGov_KpNegCurrLo_mp/1 -> BC/17  "testSig_EISGov_KpNegCurrLo_mp"
  spec_EISGov_PWinPosLo/1 -> BC/18  "testSig_EISGov_PWinPosLo"
  spec_EISGov_PWinNegLo/1 -> BC/19  "testSig_EISGov_PWinNegLo"
  spec_EISGov_KiCurrLo_mp/1 -> BC/20  "testSig_EISGov_KiCurrLo_mp"
  spec_EISGov_KiPosCurrLo_mp/1 -> BC/21  "testSig_EISGov_KiPosCurrLo_mp"
  spec_EISGov_KiNegCurrLo_mp/1 -> BC/22  "testSig_EISGov_KiNegCurrLo_mp"
  spec_EISGov_IWinPosLo/1 -> BC/23  "testSig_EISGov_IWinPosLo"
  spec_EISGov_IWinNegLo/1 -> BC/24  "testSig_EISGov_IWinNegLo"
  spec_EISGov_trqLimMin/1 -> BC/25  "testSig_EISGov_trqLimMin"
  spec_EISGov_trqLimMax/1 -> BC/26  "testSig_EISGov_trqLimMax"
  spec_EISGov_nSetPLo/1 -> BC/27  "testSig_EISGov_nSetPLo"
  spec_EISGov_nSetPHi/1 -> BC/28  "testSig_EISGov_nSetPHi"
  spec_CEngDsT_t/1 -> BC/29  "testSig_CEngDsT_t"
  spec_Oil_tSwmp/1 -> BC/30  "testSig_Oil_tSwmp"
  spec_EngDa_tEng/1 -> BC/31  "testSig_EngDa_tEng"
  spec_EISGov_numCurrFunc/1 -> BC/32  "testSig_EISGov_numCurrFunc"
  spec_EISGov_trqReq/1 -> BC/33  "testSig_EISGov_trqReq"
  spec_Epm_dnEng/1 -> BC/34  "testSig_Epm_dnEng"
  spec_EISGov_trqLosFlt/1 -> BC/35  "testSig_EISGov_trqLosFlt"
  spec_RngMod_trqCrSMin/1 -> BC/36  "testSig_RngMod_trqCrSMin"
  spec_EpmSyn_stSync/1 -> BC/37  "testSig_EpmSyn_stSync"
  spec_CoETS_stTSEATrqSpdReq/1 -> BC/38  "testSig_CoETS_stTSEATrqSpdReq"
  spec_EngDa_tStrt/1 -> BC/39  "testSig_EngDa_tStrt"
  spec_CoEng_tiNormal/1 -> BC/40  "testSig_CoEng_tiNormal"
  spec_EISGov_trqPLo/1 -> BC/41  "testSig_EISGov_trqPLo"
  spec_EISGov_trq/1 -> BC/42  "testSig_EISGov_trq"
  spec_EISGov_trqFlt/1 -> BC/43  "testSig_EISGov_trqFlt"
  spec_SpdGov_trqFlt/1 -> BC/44  "testSig_SpdGov_trqFlt"
  spec_SpdGov_trqSet/1 -> BC/45  "testSig_SpdGov_trqSet"
  spec_SpdGov_trqLead/1 -> BC/46  "testSig_SpdGov_trqLead"

== system TST_EISGov_Governor/compareSignals/Requirement_001/specifyOutputs ==
  sig_Req_Bus : Inport
  sig_Result_Bus : Inport  Port=2
  AndN : Logic  Inputs=6
  BS_Req : BusSelector  OutputSignals=testSig_EISGov_trqPLo,testSig_EISGov_trq,testSig_EISGov_trqFlt,testSig_SpdGov_trqFlt,testSig_SpdGov_trqSet,testSig_SpdGov_trqLead
  BS_Result : BusSelector  OutputSignals=EISGov_trqPLo,EISGov_trq,EISGov_trqFlt,SpdGov_trqFlt,SpdGov_trqSet,SpdGov_trqLead
  Bitwise_And{1..6} (6 alike) : simulink/Logic and Bit Operations/Bitwise Operator  logicop=AND  UseBitMask=off  BitMask=bin2dec('11011001')  BitMaskRealWorld=Stored Integer
  Scope : Scope  NumInputPorts=6
  Scope{1..6} (6 alike) : Scope  NumInputPorts=2
  cmp_{1..6} (6 alike) : UnitTest_Lib/RoughlyEqual  slope=0.1
  result_tws : ToWorkspace  VariableName=spec_result_001
  tws_1 : ToWorkspace  VariableName=spec_req_001_001
  tws_2 : ToWorkspace  VariableName=spec_req_001_002
  tws_3 : ToWorkspace  VariableName=spec_req_001_003
  tws_4 : ToWorkspace  VariableName=spec_req_001_004
  tws_5 : ToWorkspace  VariableName=spec_req_001_005
  tws_6 : ToWorkspace  VariableName=spec_req_001_006
  result : Outport
  wires:
  sig_Req_Bus/1 -> BS_Req/1
  sig_Result_Bus/1 -> BS_Result/1
  AndN/1 -> result/1, result_tws/1
  BS_Req/1 -> cmp_1/1, Scope1/1  "<testSig_EISGov_trqPLo>"
  BS_Result/1 -> cmp_1/2, Scope1/2  "<EISGov_trqPLo>"
  cmp_1/1 -> Bitwise_And1/1
  Bitwise_And1/1 -> tws_1/1, AndN/1, Scope/1
  BS_Req/2 -> cmp_2/1, Scope2/1  "<testSig_EISGov_trq>"
  BS_Result/2 -> cmp_2/2, Scope2/2  "<EISGov_trq>"
  cmp_2/1 -> Bitwise_And2/1
  Bitwise_And2/1 -> tws_2/1, AndN/2, Scope/2
  BS_Req/3 -> cmp_3/1, Scope3/1  "<testSig_EISGov_trqFlt>"
  BS_Result/3 -> cmp_3/2, Scope3/2  "<EISGov_trqFlt>"
  cmp_3/1 -> Bitwise_And3/1
  Bitwise_And3/1 -> tws_3/1, AndN/3, Scope/3
  BS_Req/4 -> cmp_4/1, Scope4/1  "<testSig_SpdGov_trqFlt>"
  BS_Result/4 -> cmp_4/2, Scope4/2  "<SpdGov_trqFlt>"
  cmp_4/1 -> Bitwise_And4/1
  Bitwise_And4/1 -> tws_4/1, AndN/4, Scope/4
  BS_Req/5 -> cmp_5/1, Scope5/1  "<testSig_SpdGov_trqSet>"
  BS_Result/5 -> cmp_5/2, Scope5/2  "<SpdGov_trqSet>"
  cmp_5/1 -> Bitwise_And5/1
  Bitwise_And5/1 -> tws_5/1, AndN/5, Scope/5
  BS_Req/6 -> cmp_6/1, Scope6/1  "<testSig_SpdGov_trqLead>"
  BS_Result/6 -> cmp_6/2, Scope6/2  "<SpdGov_trqLead>"
  cmp_6/1 -> Bitwise_And6/1
  Bitwise_And6/1 -> tws_6/1, AndN/6, Scope/6

== system TST_EISGov_Governor/compareSignals/Requirement_002/specifyOutputs ==
  sig_Req_Bus : Inport
  sig_Result_Bus : Inport  Port=2
  AndN : Logic  Inputs=6
  BS_Req : BusSelector  OutputSignals=testSig_EISGov_trqPLo,testSig_EISGov_trq,testSig_EISGov_trqFlt,testSig_SpdGov_trqFlt,testSig_SpdGov_trqSet,testSig_SpdGov_trqLead
  BS_Result : BusSelector  OutputSignals=EISGov_trqPLo,EISGov_trq,EISGov_trqFlt,SpdGov_trqFlt,SpdGov_trqSet,SpdGov_trqLead
  Bitwise_And{1..6} (6 alike) : simulink/Logic and Bit Operations/Bitwise Operator  logicop=AND  UseBitMask=off  BitMask=bin2dec('11011001')  BitMaskRealWorld=Stored Integer
  Scope : Scope  NumInputPorts=6
  Scope{1..6} (6 alike) : Scope  NumInputPorts=2
  cmp_{1..6} (6 alike) : UnitTest_Lib/RoughlyEqual  slope=0.1
  result_tws : ToWorkspace  VariableName=spec_result_002
  tws_1 : ToWorkspace  VariableName=spec_req_002_001
  tws_2 : ToWorkspace  VariableName=spec_req_002_002
  tws_3 : ToWorkspace  VariableName=spec_req_002_003
  tws_4 : ToWorkspace  VariableName=spec_req_002_004
  tws_5 : ToWorkspace  VariableName=spec_req_002_005
  tws_6 : ToWorkspace  VariableName=spec_req_002_006
  result : Outport
  wires:
  sig_Req_Bus/1 -> BS_Req/1
  sig_Result_Bus/1 -> BS_Result/1
  AndN/1 -> result/1, result_tws/1
  BS_Req/1 -> cmp_1/1, Scope1/1  "<testSig_EISGov_trqPLo>"
  BS_Result/1 -> cmp_1/2, Scope1/2  "<EISGov_trqPLo>"
  cmp_1/1 -> Bitwise_And1/1
  Bitwise_And1/1 -> tws_1/1, AndN/1, Scope/1
  BS_Req/2 -> cmp_2/1, Scope2/1  "<testSig_EISGov_trq>"
  BS_Result/2 -> cmp_2/2, Scope2/2  "<EISGov_trq>"
  cmp_2/1 -> Bitwise_And2/1
  Bitwise_And2/1 -> tws_2/1, AndN/2, Scope/2
  BS_Req/3 -> cmp_3/1, Scope3/1  "<testSig_EISGov_trqFlt>"
  BS_Result/3 -> cmp_3/2, Scope3/2  "<EISGov_trqFlt>"
  cmp_3/1 -> Bitwise_And3/1
  Bitwise_And3/1 -> tws_3/1, AndN/3, Scope/3
  BS_Req/4 -> cmp_4/1, Scope4/1  "<testSig_SpdGov_trqFlt>"
  BS_Result/4 -> cmp_4/2, Scope4/2  "<SpdGov_trqFlt>"
  cmp_4/1 -> Bitwise_And4/1
  Bitwise_And4/1 -> tws_4/1, AndN/4, Scope/4
  BS_Req/5 -> cmp_5/1, Scope5/1  "<testSig_SpdGov_trqSet>"
  BS_Result/5 -> cmp_5/2, Scope5/2  "<SpdGov_trqSet>"
  cmp_5/1 -> Bitwise_And5/1
  Bitwise_And5/1 -> tws_5/1, AndN/5, Scope/5
  BS_Req/6 -> cmp_6/1, Scope6/1  "<testSig_SpdGov_trqLead>"
  BS_Result/6 -> cmp_6/2, Scope6/2  "<SpdGov_trqLead>"
  cmp_6/1 -> Bitwise_And6/1
  Bitwise_And6/1 -> tws_6/1, AndN/6, Scope/6

== system TST_EISGov_Governor/compareSignals/Requirement_003/specifyOutputs ==
  sig_Req_Bus : Inport
  sig_Result_Bus : Inport  Port=2
  AndN : Logic  Inputs=6
  BS_Req : BusSelector  OutputSignals=testSig_EISGov_trqPLo,testSig_EISGov_trq,testSig_EISGov_trqFlt,testSig_SpdGov_trqFlt,testSig_SpdGov_trqSet,testSig_SpdGov_trqLead
  BS_Result : BusSelector  OutputSignals=EISGov_trqPLo,EISGov_trq,EISGov_trqFlt,SpdGov_trqFlt,SpdGov_trqSet,SpdGov_trqLead
  Bitwise_And{1..6} (6 alike) : simulink/Logic and Bit Operations/Bitwise Operator  logicop=AND  UseBitMask=off  BitMask=bin2dec('11011001')  BitMaskRealWorld=Stored Integer
  Scope : Scope  NumInputPorts=6
  Scope{1..6} (6 alike) : Scope  NumInputPorts=2
  cmp_{1..6} (6 alike) : UnitTest_Lib/RoughlyEqual  slope=0.1
  result_tws : ToWorkspace  VariableName=spec_result_003
  tws_1 : ToWorkspace  VariableName=spec_req_003_001
  tws_2 : ToWorkspace  VariableName=spec_req_003_002
  tws_3 : ToWorkspace  VariableName=spec_req_003_003
  tws_4 : ToWorkspace  VariableName=spec_req_003_004
  tws_5 : ToWorkspace  VariableName=spec_req_003_005
  tws_6 : ToWorkspace  VariableName=spec_req_003_006
  result : Outport
  wires:
  sig_Req_Bus/1 -> BS_Req/1
  sig_Result_Bus/1 -> BS_Result/1
  AndN/1 -> result/1, result_tws/1
  BS_Req/1 -> cmp_1/1, Scope1/1  "<testSig_EISGov_trqPLo>"
  BS_Result/1 -> cmp_1/2, Scope1/2  "<EISGov_trqPLo>"
  cmp_1/1 -> Bitwise_And1/1
  Bitwise_And1/1 -> tws_1/1, AndN/1, Scope/1
  BS_Req/2 -> cmp_2/1, Scope2/1  "<testSig_EISGov_trq>"
  BS_Result/2 -> cmp_2/2, Scope2/2  "<EISGov_trq>"
  cmp_2/1 -> Bitwise_And2/1
  Bitwise_And2/1 -> tws_2/1, AndN/2, Scope/2
  BS_Req/3 -> cmp_3/1, Scope3/1  "<testSig_EISGov_trqFlt>"
  BS_Result/3 -> cmp_3/2, Scope3/2  "<EISGov_trqFlt>"
  cmp_3/1 -> Bitwise_And3/1
  Bitwise_And3/1 -> tws_3/1, AndN/3, Scope/3
  BS_Req/4 -> cmp_4/1, Scope4/1  "<testSig_SpdGov_trqFlt>"
  BS_Result/4 -> cmp_4/2, Scope4/2  "<SpdGov_trqFlt>"
  cmp_4/1 -> Bitwise_And4/1
  Bitwise_And4/1 -> tws_4/1, AndN/4, Scope/4
  BS_Req/5 -> cmp_5/1, Scope5/1  "<testSig_SpdGov_trqSet>"
  BS_Result/5 -> cmp_5/2, Scope5/2  "<SpdGov_trqSet>"
  cmp_5/1 -> Bitwise_And5/1
  Bitwise_And5/1 -> tws_5/1, AndN/5, Scope/5
  BS_Req/6 -> cmp_6/1, Scope6/1  "<testSig_SpdGov_trqLead>"
  BS_Result/6 -> cmp_6/2, Scope6/2  "<SpdGov_trqLead>"
  cmp_6/1 -> Bitwise_And6/1
  Bitwise_And6/1 -> tws_6/1, AndN/6, Scope/6

== system TST_EISGov_Governor/compareSignals/Requirement_004/specifyOutputs ==
  sig_Req_Bus : Inport
  sig_Result_Bus : Inport  Port=2
  AndN : Logic  Inputs=6
  BS_Req : BusSelector  OutputSignals=testSig_EISGov_trqPLo,testSig_EISGov_trq,testSig_EISGov_trqFlt,testSig_SpdGov_trqFlt,testSig_SpdGov_trqSet,testSig_SpdGov_trqLead
  BS_Result : BusSelector  OutputSignals=EISGov_trqPLo,EISGov_trq,EISGov_trqFlt,SpdGov_trqFlt,SpdGov_trqSet,SpdGov_trqLead
  Bitwise_And{1..6} (6 alike) : simulink/Logic and Bit Operations/Bitwise Operator  logicop=AND  UseBitMask=off  BitMask=bin2dec('11011001')  BitMaskRealWorld=Stored Integer
  Scope : Scope  NumInputPorts=6
  Scope{1..6} (6 alike) : Scope  NumInputPorts=2
  cmp_{1..6} (6 alike) : UnitTest_Lib/RoughlyEqual  slope=0.1
  result_tws : ToWorkspace  VariableName=spec_result_004
  tws_1 : ToWorkspace  VariableName=spec_req_004_001
  tws_2 : ToWorkspace  VariableName=spec_req_004_002
  tws_3 : ToWorkspace  VariableName=spec_req_004_003
  tws_4 : ToWorkspace  VariableName=spec_req_004_004
  tws_5 : ToWorkspace  VariableName=spec_req_004_005
  tws_6 : ToWorkspace  VariableName=spec_req_004_006
  result : Outport
  wires:
  sig_Req_Bus/1 -> BS_Req/1
  sig_Result_Bus/1 -> BS_Result/1
  AndN/1 -> result/1, result_tws/1
  BS_Req/1 -> cmp_1/1, Scope1/1  "<testSig_EISGov_trqPLo>"
  BS_Result/1 -> cmp_1/2, Scope1/2  "<EISGov_trqPLo>"
  cmp_1/1 -> Bitwise_And1/1
  Bitwise_And1/1 -> tws_1/1, AndN/1, Scope/1
  BS_Req/2 -> cmp_2/1, Scope2/1  "<testSig_EISGov_trq>"
  BS_Result/2 -> cmp_2/2, Scope2/2  "<EISGov_trq>"
  cmp_2/1 -> Bitwise_And2/1
  Bitwise_And2/1 -> tws_2/1, AndN/2, Scope/2
  BS_Req/3 -> cmp_3/1, Scope3/1  "<testSig_EISGov_trqFlt>"
  BS_Result/3 -> cmp_3/2, Scope3/2  "<EISGov_trqFlt>"
  cmp_3/1 -> Bitwise_And3/1
  Bitwise_And3/1 -> tws_3/1, AndN/3, Scope/3
  BS_Req/4 -> cmp_4/1, Scope4/1  "<testSig_SpdGov_trqFlt>"
  BS_Result/4 -> cmp_4/2, Scope4/2  "<SpdGov_trqFlt>"
  cmp_4/1 -> Bitwise_And4/1
  Bitwise_And4/1 -> tws_4/1, AndN/4, Scope/4
  BS_Req/5 -> cmp_5/1, Scope5/1  "<testSig_SpdGov_trqSet>"
  BS_Result/5 -> cmp_5/2, Scope5/2  "<SpdGov_trqSet>"
  cmp_5/1 -> Bitwise_And5/1
  Bitwise_And5/1 -> tws_5/1, AndN/5, Scope/5
  BS_Req/6 -> cmp_6/1, Scope6/1  "<testSig_SpdGov_trqLead>"
  BS_Result/6 -> cmp_6/2, Scope6/2  "<SpdGov_trqLead>"
  cmp_6/1 -> Bitwise_And6/1
  Bitwise_And6/1 -> tws_6/1, AndN/6, Scope/6

== system TST_EISGov_Governor/compareSignals/Requirement_005/specifyOutputs ==
  sig_Req_Bus : Inport
  sig_Result_Bus : Inport  Port=2
  AndN : Logic  Inputs=6
  BS_Req : BusSelector  OutputSignals=testSig_EISGov_trqPLo,testSig_EISGov_trq,testSig_EISGov_trqFlt,testSig_SpdGov_trqFlt,testSig_SpdGov_trqSet,testSig_SpdGov_trqLead
  BS_Result : BusSelector  OutputSignals=EISGov_trqPLo,EISGov_trq,EISGov_trqFlt,SpdGov_trqFlt,SpdGov_trqSet,SpdGov_trqLead
  Bitwise_And{1..6} (6 alike) : simulink/Logic and Bit Operations/Bitwise Operator  logicop=AND  UseBitMask=off  BitMask=bin2dec('11011001')  BitMaskRealWorld=Stored Integer
  Scope : Scope  NumInputPorts=6
  Scope{1..6} (6 alike) : Scope  NumInputPorts=2
  cmp_{1..6} (6 alike) : UnitTest_Lib/RoughlyEqual  slope=0.1
  result_tws : ToWorkspace  VariableName=spec_result_005
  tws_1 : ToWorkspace  VariableName=spec_req_005_001
  tws_2 : ToWorkspace  VariableName=spec_req_005_002
  tws_3 : ToWorkspace  VariableName=spec_req_005_003
  tws_4 : ToWorkspace  VariableName=spec_req_005_004
  tws_5 : ToWorkspace  VariableName=spec_req_005_005
  tws_6 : ToWorkspace  VariableName=spec_req_005_006
  result : Outport
  wires:
  sig_Req_Bus/1 -> BS_Req/1
  sig_Result_Bus/1 -> BS_Result/1
  AndN/1 -> result/1, result_tws/1
  BS_Req/1 -> cmp_1/1, Scope1/1  "<testSig_EISGov_trqPLo>"
  BS_Result/1 -> cmp_1/2, Scope1/2  "<EISGov_trqPLo>"
  cmp_1/1 -> Bitwise_And1/1
  Bitwise_And1/1 -> tws_1/1, AndN/1, Scope/1
  BS_Req/2 -> cmp_2/1, Scope2/1  "<testSig_EISGov_trq>"
  BS_Result/2 -> cmp_2/2, Scope2/2  "<EISGov_trq>"
  cmp_2/1 -> Bitwise_And2/1
  Bitwise_And2/1 -> tws_2/1, AndN/2, Scope/2
  BS_Req/3 -> cmp_3/1, Scope3/1  "<testSig_EISGov_trqFlt>"
  BS_Result/3 -> cmp_3/2, Scope3/2  "<EISGov_trqFlt>"
  cmp_3/1 -> Bitwise_And3/1
  Bitwise_And3/1 -> tws_3/1, AndN/3, Scope/3
  BS_Req/4 -> cmp_4/1, Scope4/1  "<testSig_SpdGov_trqFlt>"
  BS_Result/4 -> cmp_4/2, Scope4/2  "<SpdGov_trqFlt>"
  cmp_4/1 -> Bitwise_And4/1
  Bitwise_And4/1 -> tws_4/1, AndN/4, Scope/4
  BS_Req/5 -> cmp_5/1, Scope5/1  "<testSig_SpdGov_trqSet>"
  BS_Result/5 -> cmp_5/2, Scope5/2  "<SpdGov_trqSet>"
  cmp_5/1 -> Bitwise_And5/1
  Bitwise_And5/1 -> tws_5/1, AndN/5, Scope/5
  BS_Req/6 -> cmp_6/1, Scope6/1  "<testSig_SpdGov_trqLead>"
  BS_Result/6 -> cmp_6/2, Scope6/2  "<SpdGov_trqLead>"
  cmp_6/1 -> Bitwise_And6/1
  Bitwise_And6/1 -> tws_6/1, AndN/6, Scope/6
